simulink subsystem "s3EMSSC"  (R2023b)
settings: Solver=VariableStepAuto  StartTime=0.0  StopTime=10.0  RelTol=1e-3
undefined symbols (not defined in the file): EM1, EM2, EM3, ThrmEM1, ThrmEM2, ThrmEM3
settings Model: Creator=The MathWorks, Inc.  LastModifiedBy=The MathWorks, Inc.

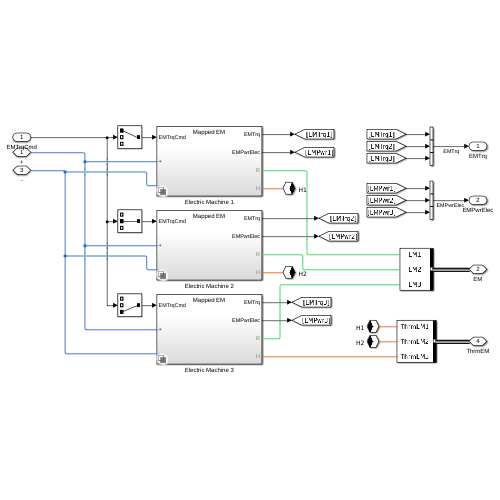
[thumbnail: Simulink's stored preview of the top-level diagram]
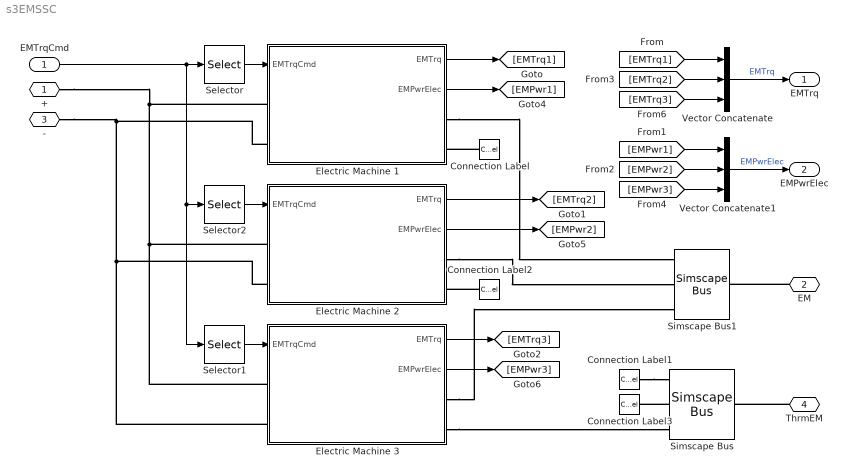
== system s3EMSSC ==
  EMTrqCmd : Inport
  Connection Label : ConnectionLabel  Label=H1
  Connection Label1 : ConnectionLabel  Label=H1
  Connection Label2 : ConnectionLabel  Label=H2
  Connection Label3 : ConnectionLabel  Label=H2
  Electric Machine 1 : Subsystem  Variant=on  VariantControlMode=label  LabelModeActiveChoice=Mapped EM
  Electric Machine 2 : Subsystem  Variant=on  VariantControlMode=label  LabelModeActiveChoice=Mapped EM
  Electric Machine 3 : Subsystem  Variant=on  VariantControlMode=label  LabelModeActiveChoice=Mapped EM
  Selector : Selector  InputPortWidth=3  IndexOptions=Index vector (dialog)  Indices=[1]  OutputSizes=1
  Selector1 : Selector  InputPortWidth=3  IndexOptions=Index vector (dialog)  Indices=[3]  OutputSizes=1
  Selector2 : Selector  InputPortWidth=3  IndexOptions=Index vector (dialog)  Indices=[2]  OutputSizes=1
  Simscape Bus : SimscapeBus  HierarchyStrings=ThrmEM1;ThrmEM2;ThrmEM3
  Simscape Bus1 : SimscapeBus  HierarchyStrings=EM1;EM2;EM3
  Vector Concatenate : Concatenate  NumInputs=3
  Vector Concatenate1 : Concatenate  NumInputs=3
  + : PMIOPort  Side=Left
  EM : PMIOPort  Port=2  Side=Right
  - : PMIOPort  Port=3  Side=Left
  ThrmEM : PMIOPort  Port=4  Side=Right
  EMTrq : Outport
  EMPwrElec : Outport  Port=2
  wires:
  Selector/1 -> Electric Machine 1/1(EMTrqCmd)
  EMTrqCmd/1 -> Selector1/1, Selector2/1, Selector/1
  Vector Concatenate/1 -> EMTrq/1  "EMTrq"
  Vector Concatenate1/1 -> EMPwrElec/1  "EMPwrElec"
  Selector2/1 -> Electric Machine 2/1(EMTrqCmd)
  Selector1/1 -> Electric Machine 3/1(EMTrqCmd)
  Electric Machine 1/1(EMTrq) -> [EMTrq1]
  [EMTrq1] -> Vector Concatenate/1
  [EMTrq2] -> Vector Concatenate/2
  [EMTrq3] -> Vector Concatenate/3
  Electric Machine 2/1(EMTrq) -> [EMTrq2]
  Electric Machine 3/1(EMTrq) -> [EMTrq3]
  Electric Machine 1/2(EMPwrElec) -> [EMPwr1]
  [EMPwr1] -> Vector Concatenate1/1
  Electric Machine 2/2(EMPwrElec) -> [EMPwr2]
  [EMPwr2] -> Vector Concatenate1/2
  Electric Machine 3/2(EMPwrElec) -> [EMPwr3]
  [EMPwr3] -> Vector Concatenate1/3
  connections:
  Electric Machine 2/LConn2 -- Electric Machine 3/LConn2 -- -/RConn1 -- Electric Machine 1/LConn2
  Electric Machine 2/LConn1 -- Electric Machine 3/LConn1 -- +/RConn1 -- Electric Machine 1/LConn1
  Electric Machine 3/RConn2 -- Simscape Bus/LConn3
  Connection Label2/LConn1 -- Electric Machine 2/RConn2
  Connection Label/LConn1 -- Electric Machine 1/RConn2
  ThrmEM/RConn1 -- Simscape Bus/RConn1
  Simscape Bus/LConn2 -- Connection Label3/LConn1
  Connection Label1/LConn1 -- Simscape Bus/LConn1
  Electric Machine 1/RConn1 -- Simscape Bus1/LConn1
  Electric Machine 2/RConn1 -- Simscape Bus1/LConn2
  EM/RConn1 -- Simscape Bus1/RConn1
  Electric Machine 3/RConn1 -- Simscape Bus1/LConn3

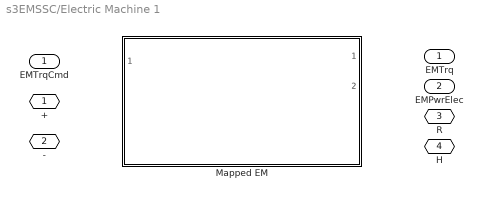
== system s3EMSSC/Electric Machine 1 ==
  EMTrqCmd : Inport
  Mapped EM : Subsystem  VariantControl=Mapped EM  ReferencedSubsystem=ElectricMachine1SSC
  + : PMIOPort  Side=Left
  - : PMIOPort  Port=2  Side=Left
  R : PMIOPort  Port=3  Side=Right
  H : PMIOPort  Port=4  Side=Right
  EMTrq : Outport  VectorParamsAs1DForOutWhenUnconnected=off
  EMPwrElec : Outport  Port=2  VectorParamsAs1DForOutWhenUnconnected=off

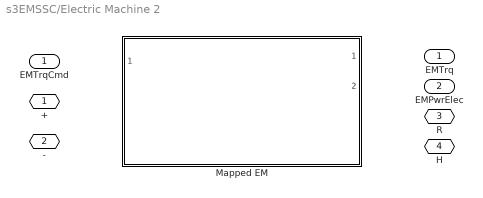
== system s3EMSSC/Electric Machine 2 ==
  EMTrqCmd : Inport
  Mapped EM : Subsystem  VariantControl=Mapped EM  ReferencedSubsystem=ElectricMachine2SSC
  + : PMIOPort  Side=Left
  - : PMIOPort  Port=2  Side=Left
  R : PMIOPort  Port=3  Side=Right
  H : PMIOPort  Port=4  Side=Right
  EMTrq : Outport  VectorParamsAs1DForOutWhenUnconnected=off
  EMPwrElec : Outport  Port=2  VectorParamsAs1DForOutWhenUnconnected=off

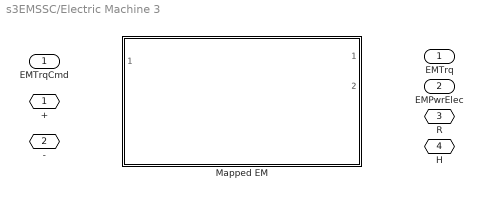
== system s3EMSSC/Electric Machine 3 ==
  EMTrqCmd : Inport
  Mapped EM : Subsystem  VariantControl=Mapped EM  ReferencedSubsystem=ElectricMachine3SSC
  + : PMIOPort  Side=Left
  - : PMIOPort  Port=2  Side=Left
  R : PMIOPort  Port=3  Side=Right
  H : PMIOPort  Port=4  Side=Right
  EMTrq : Outport  VectorParamsAs1DForOutWhenUnconnected=off
  EMPwrElec : Outport  Port=2  VectorParamsAs1DForOutWhenUnconnected=off
